simulink model "mpc_CSTR"  (R2017a)
settings: Solver=ode23  StartTime=0.0  StopTime=0.03  RelTol=1e-3
values from neighbouring files (symbols this model uses):
  Ap = [-1/(R*C)   1/C        0    -1/C      1/C        0 ... (first row only)    [GeneradoresInterconectados.m]
  Bp = [    0      0 ... (first row only)    [GeneradoresInterconectados.m]
  Cp = [    1      0 ... (first row only)    [GeneradoresInterconectados.m]
  Dp = zeros(2,2)    [GeneradoresInterconectados.m]
  I2 = 18    [GeneradoresInterconectados.m]
  R = 1000    [GeneradoresInterconectados.m]
undefined symbols (not defined in the file or in its folder): I1
libraries: mpclib x1, powerlib x1
settings Model: ExtModeTrigMode=oneshot  ExtModeArmWhenConnect=off  Creator=The MathWorks Inc.  LastModifiedBy=Administrador
settings DataIOCC: SaveFormat=Array  SaveOutput=off  SignalLogging=off  DSMLogging=off  SaveTime=off  SignalLoggingName=sigsOut
settings OptimizationCC: BooleanDataType=off  ExpressionDepthLimit=2147483647  InitFltsAndDblsToZero=on  LifeSpan=inf
settings DebuggingCC: SaveWithParameterizedLinksMsg=none  UnderspecifiedInitializationDetection=Classic  MergeDetectMultiDrivingBlocksExec=none  SignalResolutionControl=TryResolveAllWithWarning  MultiTaskDSMMsg=warning  MultiTaskCondExecSysMsg=none  IntegerOverflowMsg=none  FcnCallInpInsideContextMsg=warning  StateNameClashWarn=warning  SFUnexpectedBacktrackingDiag=warning  SFNoUnconditionalDefaultTransitionDiag=warning  SFExecutionAtInitializationDiag=none  IntegerSaturationMsg=none
settings HardwareCC: ProdBitPerPointer=32  ProdBitPerSizeT=32  ProdBitPerPtrDiffT=32  ProdLargestAtomicFloat=None  ProdIntDivRoundTo=Undefined  ProdEndianess=Unspecified  ProdWordSize=32  ProdHWDeviceType=32-bit Generic  TargetUnknown=on
settings ModelReferenceCC: PropagateSignalLabelsOutOfModel=off
settings GRTTargetCC: TargetFcnLib=ansi_tfl_tmw.mat  TargetLangStandard=C89/C90 (ANSI)  GeneratePreprocessorConditionals=Disable all  CombineOutputUpdateFcns=off  GRTInterface=on
settings ConfigComp: CovMetricSettings=dw  CovHtmlReporting=on  CovSaveCumulativeToWorkspaceVar=on  CovSaveSingleToWorkspaceVar=on  CovExternalEMLEnable=off  CovSFcnEnable=off

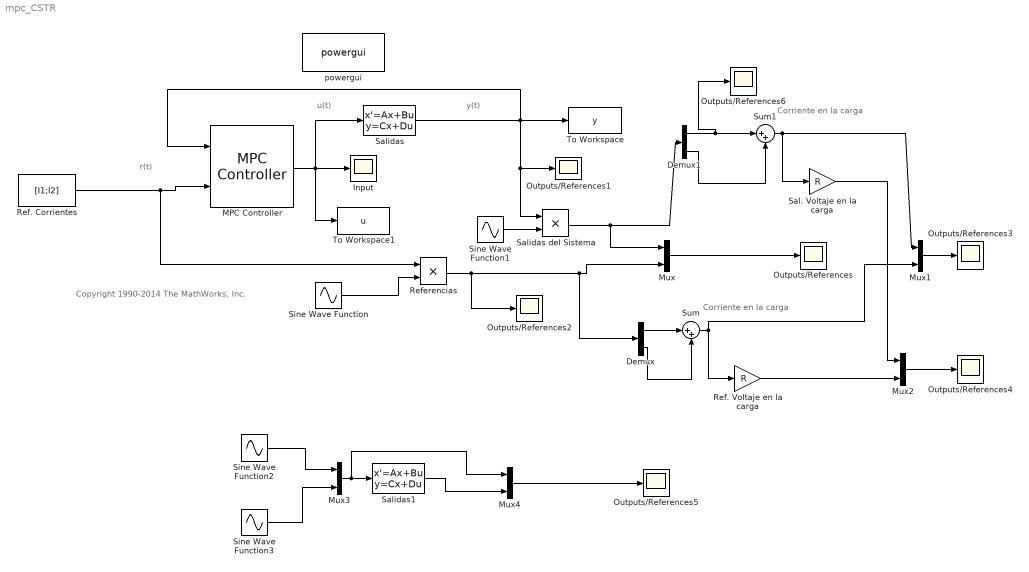
== system mpc_CSTR ==
  note: Corriente en la carga
  note: u(t)
  note: y(t)
  note: r(t)
  note: Copyright 1990-2014 The MathWorks, Inc.
  note: Corriente en la carga
  Demux : Demux  Outputs=2
  Demux1 : Demux  Outputs=2
  Input : Scope
  MPC Controller : mpclib/MPC Controller  mpcobj=mpcobj  x0=[]  is_multiple=0  enable_value=0  return_u0=off  ref_from_ws=off  ref_signal_name=[]  ref_preview=on  md_from_ws=off  md_signal_name=[]  md_preview=on  from_project=off  project_file=MPCtask.mat  md_inport=off  mv_inport=off  cost_outport=off  return_sequence=off  return_qpstatus=off  return_state=off  state_inport=off  lims_inport=off  ywt_inport=off  is_designfromscratch=0  uwt_inport=off  duwt_inport=off  rhoeps_inport=off  uref_inport=off  n_ts=0.1  n_mv=2  n_md=0  n_ud=0  n_mo=2  n_uo=0  BlockDataType=double  SampleTimeInherited=off  switch_inport=off
  Mux{,1..4} (5 alike) : Mux  Inputs=2
  Outputs/References{,1..6} (7 alike) : Scope
  Ref. Corrientes : Constant  Value=[I1;I2]
  Ref. Voltaje en la carga : Gain  Gain=R
  Referencias : Product
  Sal. Voltaje en la carga : Gain  Gain=R
  Salidas : StateSpace  A=Ap  B=Bp  C=Cp  D=Dp  X0=0
  Salidas del Sistema : Product
  Salidas1 : StateSpace  A=Ap  B=Bp  C=Cp  D=Dp  X0=0
  Sine Wave Function : Sin  Frequency=2*pi*60  Samples=60  SampleTime=0
  Sine Wave Function1 : Sin  Frequency=2*pi*60  Samples=60  SampleTime=0
  Sine Wave Function2 : Sin  Amplitude=1.17  Frequency=2*pi*60  Samples=60  SampleTime=0
  Sine Wave Function3 : Sin  Amplitude=3  Frequency=2*pi*60  Samples=60  SampleTime=0
  Sum : Sum  Inputs=|++
  Sum1 : Sum  Inputs=|++
  To Workspace : ToWorkspace  VariableName=y  SampleTime=-1
      settings: MaxDataPoints=Inf
  To Workspace1 : ToWorkspace  VariableName=u  SampleTime=-1
      settings: MaxDataPoints=Inf
  powergui : powerlib/powergui  SimulationMode=Discrete  SampleTime=1/60/10000  frequency=60  Iterations=50  frequencyindice=0  Pbase=100e6  ErrMax=1e-4  UnitsV=kV  UnitsW=MW  buscounter=0  FunctionMessages=off  echomessages=off  EnableUseOfTLC=off  CurrentSourceSwitches=off  DisableSnubberDevices=off  DisableRonSwitches=off  DisableVfSwitches=off  DisplayEquations=off  SolverType=Tustin/Backward Euler (TBE)  Interpol=off  ExternalGateDelay=off  methode=off  Ts=100  x0status=blocks  SPID=on  SwTol=0  HookPort=off  RestoreLinks=warning  ResistiveCurrentMeasurement=off  Frange=[0:2:500]  Ylog=off  Xlog=on  ShowGrid=off  save=off  variable=ZData  structure=sps1phPWM1_str  ZoomFFT=on  StartTime=0.1-2/60  cycles=2  DisplayStyle=1  fundamental=60  FreqAxis=off  MaxFrequency=5000  frequencyindicesteady=1  RmsSteady=1  display=off
  wires:
  MPC Controller/1 -> Salidas/1, Input/1, To Workspace1/1
  Salidas/1 -> To Workspace/1, Salidas del Sistema/1, Outputs/References1/1, MPC Controller/1
  Ref. Corrientes/1 -> Referencias/1, MPC Controller/2
  Sine Wave Function/1 -> Referencias/2
  Sine Wave Function1/1 -> Salidas del Sistema/2
  Salidas del Sistema/1 -> Demux1/1, Mux/1
  Referencias/1 -> Outputs/References2/1, Demux/1, Mux/2
  Mux/1 -> Outputs/References/1
  Demux/1 -> Sum/1
  Demux/2 -> Sum/2
  Sum/1 -> Ref. Voltaje en la carga/1, Mux1/2
  Sum1/1 -> Mux1/1, Sal. Voltaje en la carga/1
  Sal. Voltaje en la carga/1 -> Mux2/1
  Demux1/2 -> Sum1/2
  Demux1/1 -> Outputs/References6/1, Sum1/1
  Mux1/1 -> Outputs/References3/1
  Ref. Voltaje en la carga/1 -> Mux2/2
  Mux2/1 -> Outputs/References4/1
  Sine Wave Function2/1 -> Mux3/1
  Sine Wave Function3/1 -> Mux3/2
  Mux4/1 -> Outputs/References5/1
  Salidas1/1 -> Mux4/2
  Mux3/1 -> Mux4/1, Salidas1/1
